simulink model "PMSM"  (R2024b)
settings: Solver=VariableStepAuto  StartTime=0.0  StopTime=3  RelTol=1e-3
values from neighbouring files (symbols this model uses):
  f_peak = 60    [PMSM_machine.m]
  J_total = 340e-6    (= 0.00034)    [PMSM_machine.m]
  Ls = 1365e-6    (= 0.001365)    [PMSM_machine.m]
  p = 2    [PMSM_machine.m]
  Psi_f = 0.166    [PMSM_machine.m]
  Rs = 0.416    [PMSM_machine.m]
  T_nom = 10    [PMSM_machine.m]
  t_ramp = 0.5    [PMSM_machine.m]
  U_peak = 60    [PMSM_machine.m]
libraries: mcbcontrolslib x4, simulink x2, eeTransforms x1
settings Model: Creator=chinm  LastModifiedBy=chinm

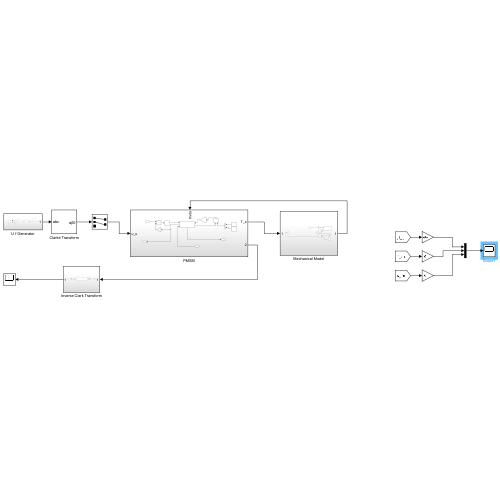
[thumbnail: Simulink's stored preview of the top-level diagram]
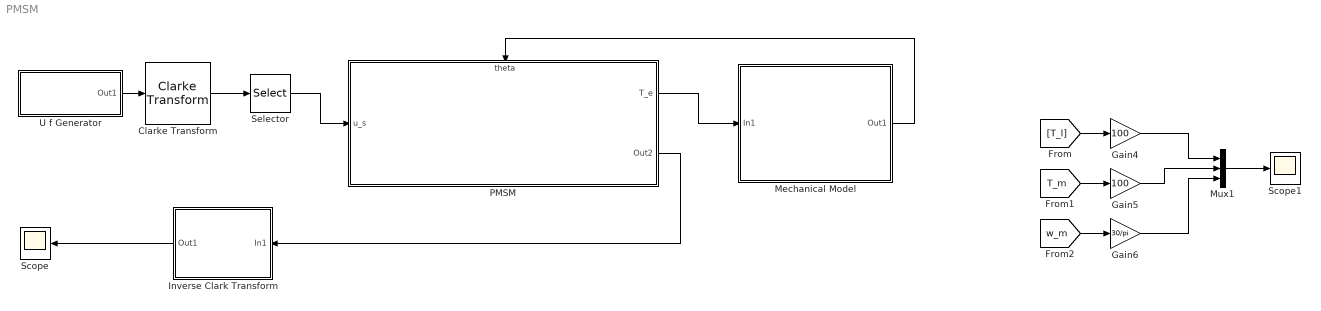
== system PMSM ==
  Clarke Transform : eeTransforms/Clarke Transform  PowerInvariant=off
      settings: LibrarySourceBlock=|
      | ee_sl_lib/Mathematical
      | Transforms/Clarke Transform
  Gain4 : Gain  Gain=100
  Gain5 : Gain  Gain=100
  Gain6 : Gain  Gain=30/pi
  Inverse Clark Transform : Subsystem
  Mechanical Model : Subsystem
  Mux1 : Mux  Inputs=3
  PMSM : Subsystem
      settings: PortSchema="{\"entries\":[{\"content\":{\"sides\":[{\"content\":{\"connectorIds\":[\"In1\"]},\"type\":\"ConnectorPlacement.EquallySpacedRectSide\",\"uuid\":\"4cb8065a-e5a2-415d-9e19-2924cebdfb7e\"},{\"content\":{\"connectorIds\":[\"Out1\",\"Out2\"],\"side\":\"RIGHT\"},\"type\":\"ConnectorPlacement.EquallySpacedRectSide\",\"uuid\":\"835c200d-c821-4b36-b5e5-04b20f8cfe15\"},{\"content\":{\"connectorIds\":[\"In2\"],\"side\":\"TOP\"},\"type\":\"ConnectorPlacement.EquallySpacedRectSide\",\"uuid\":\"b9320f7a-4b67-4ae1-910b-20da4fa2f11a\"}]},\"type\":\"ConnectorPlacement.EquallySpacedConnector\",\"uuid\":\"30be06dc-1f8c-4f24-82eb-4e3de7bbb2e4\"}],\"packageUris\":[\"http://schema.mathworks.com/mf0/Connector/R2020b\"],\"version\":\"1.0\"}"
  Scope : Scope
  Scope1 : Scope
  Selector : Selector  InputPortWidth=3  IndexOptions=Index vector (dialog)  Indices=[1 2]  OutputSizes=1
  U f Generator : Subsystem
  wires:
  U f Generator/1(Out1) -> Clarke Transform/1
  Clarke Transform/1 -> Selector/1
  Inverse Clark Transform/1(Out1) -> Scope/1
  [T_l] -> Gain4/1
  [T_m] -> Gain5/1
  [w_m] -> Gain6/1
  Mux1/1 -> Scope1/1
  Gain5/1 -> Mux1/2
  Gain4/1 -> Mux1/1
  Gain6/1 -> Mux1/3
  Selector/1 -> PMSM/1(u_s)
  PMSM/2(Out2) -> Inverse Clark Transform/1(In1)
  PMSM/1(T_e) -> Mechanical Model/1(In1)
  Mechanical Model/1(Out1) -> PMSM/2(theta)

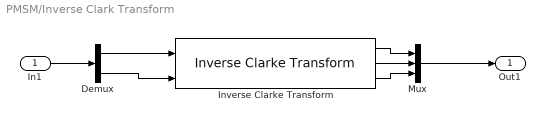
== system PMSM/Inverse Clark Transform ==
  In1 : Inport
  Demux : Demux  Outputs=2
  Inverse Clarke Transform : mcbcontrolslib/Inverse Clarke Transform  PhaseInput=Two inputs  EnPowerInv=off
      settings: LibrarySourceBlock=mcblib/Controls/Math Transforms/Inverse Clarke Transform
  Mux : Mux  Inputs=3
  Out1 : Outport
  wires:
  In1/1 -> Demux/1
  Demux/2 -> Inverse Clarke Transform/2
  Demux/1 -> Inverse Clarke Transform/1
  Inverse Clarke Transform/1 -> Mux/1
  Inverse Clarke Transform/2 -> Mux/2
  Inverse Clarke Transform/3 -> Mux/3
  Mux/1 -> Out1/1

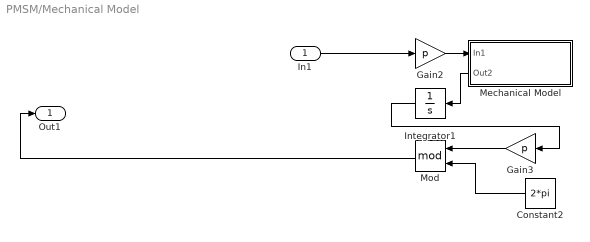
== system PMSM/Mechanical Model ==
  In1 : Inport
  Constant2 : Constant  Value=2*pi
  Gain2 : Gain  Gain=p
  Gain3 : Gain  Gain=p
  Integrator1 : Integrator
  Mechanical Model : Subsystem
      settings: PortSchema="{\"entries\":[{\"content\":{\"sides\":[{\"content\":{\"connectorIds\":[\"In1\",\"Out1\"]},\"type\":\"ConnectorPlacement.EquallySpacedRectSide\",\"uuid\":\"b4986fb2-c57d-4b73-a735-292653fff6d9\"},{\"content\":{\"side\":\"RIGHT\"},\"type\":\"ConnectorPlacement.EquallySpacedRectSide\",\"uuid\":\"9d0dc8a9-3fda-4760-870c-c4cad97d429b\"},{\"content\":{\"side\":\"TOP\"},\"type\":\"ConnectorPlacement.EquallySpacedRectSide\",\"uuid\":\"e1f646a3-730d-45a9-a867-cd53dcd150be\"}]},\"type\":\"ConnectorPlacement.EquallySpacedConnector\",\"uuid\":\"ab7f54df-393a-4b01-99b4-3432e63bf963\"}],\"packageUris\":[\"http://schema.mathworks.com/mf0/Connector/R2020b\"],\"version\":\"1.0\"}"
  Mod : Math  Operator=mod
  Out1 : Outport
  wires:
  Gain3/1 -> Mod/1
  Constant2/1 -> Mod/2
  Mechanical Model/1(Out2) -> Integrator1/1
  Integrator1/1 -> Gain3/1
  In1/1 -> Gain2/1
  Gain2/1 -> Mechanical Model/1(In1)
  Mod/1 -> Out1/1

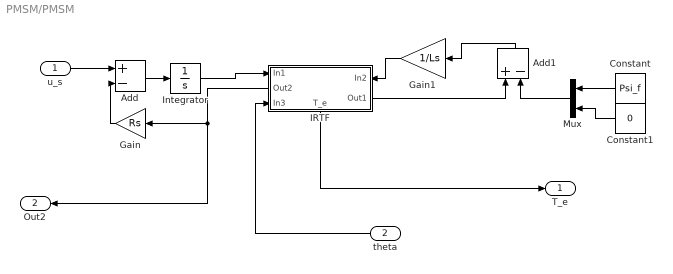
== system PMSM/PMSM ==
  u_s : Inport
  theta : Inport  Port=2
  Add : Sum  Inputs=+-
  Add1 : Sum  Inputs=+-
  Constant : Constant  Value=Psi_f
  Constant1 : Constant  Value=0
  Gain : Gain  Gain=Rs
  Gain1 : Gain  Gain=1/Ls
  IRTF : Subsystem
      settings: PortSchema="{\"entries\":[{\"content\":{\"sides\":[{\"content\":{\"connectorIds\":[\"In1\",\"Out3\",\"In2\"]},\"type\":\"ConnectorPlacement.EquallySpacedRectSide\",\"uuid\":\"b4986fb2-c57d-4b73-a735-292653fff6d9\"},{\"content\":{\"connectorIds\":[\"In3\",\"Out1\"],\"side\":\"RIGHT\"},\"type\":\"ConnectorPlacement.EquallySpacedRectSide\",\"uuid\":\"9d0dc8a9-3fda-4760-870c-c4cad97d429b\"},{\"content\":{\"side\":\"TOP\"},\"type\":\"ConnectorPlacement.EquallySpacedRectSide\",\"uuid\":\"e1f646a3-730d-45a9-a867-cd53dcd150be\"},{\"content\":{\"connectorIds\":[\"Out2\"],\"side\":\"BOTTOM\"},\"type\":\"ConnectorPlacement.EquallySpacedRectSide\",\"uuid\":\"c6f4b204-5ea6-4623-acea-3e4f968e6d8a\"}]},\"type\":\"ConnectorPlacement.EquallySpacedConnector\",\"uuid\":\"ab7f54df-393a-4b01-99b4-3432e63bf963\"}],\"packageUris\":[\"http://schema.mathworks.com/mf0/Connector/R2020b\"],\"version\":\"1.0\"}"
  Integrator : Integrator
  Mux : Mux  Inputs=2
  T_e : Outport
  Out2 : Outport  Port=2
  wires:
  IRTF/3(Out2) -> Out2/1, Gain/1
  Gain/1 -> Add/2
  u_s/1 -> Add/1
  Add/1 -> Integrator/1
  Integrator/1 -> IRTF/1(In1)
  Add1/1 -> Gain1/1
  Constant/1 -> Mux/1
  Constant1/1 -> Mux/2
  IRTF/1(Out1) -> Add1/1
  Mux/1 -> Add1/2
  Gain1/1 -> IRTF/3(In2)
  theta/1 -> IRTF/2(In3)
  IRTF/2(T_e) -> T_e/1

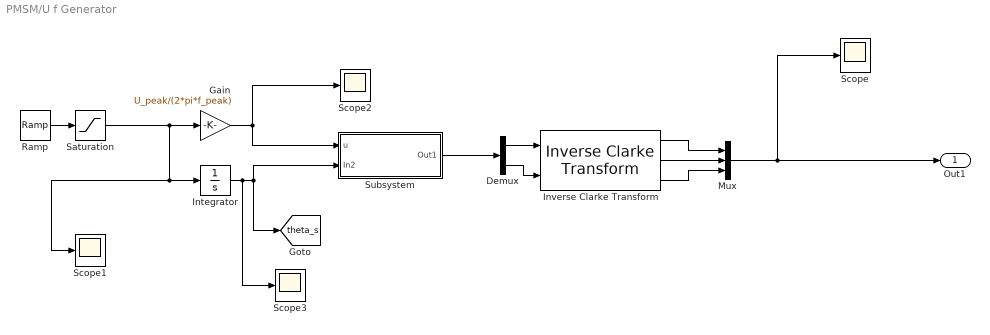
== system PMSM/U f Generator ==
  Demux : Demux  Outputs=2
  Gain : Gain  Gain=U_peak/(2*pi*f_peak)
  Integrator : Integrator  LimitOutput=on  WrappedStateUpperValue=2*pi  WrappedStateLowerValue=0  ZeroCross=off
  Inverse Clarke Transform : mcbcontrolslib/Inverse Clarke Transform  PhaseInput=Two inputs  EnPowerInv=off
      settings: LibrarySourceBlock=mcblib/Controls/Math Transforms/Inverse Clarke Transform
  Mux : Mux  Inputs=3
  Ramp : simulink/Sources/Ramp  slope=f_peak*2*pi/t_ramp  start=0  InitialOutput=0
  Saturation : Saturate  UpperLimit=2*pi*f_peak  LowerLimit=0
  Scope{,1..3} (4 alike) : Scope
  Subsystem : Subsystem
  Out1 : Outport
  tag scope: theta_s=global
  wires:
  Gain/1 -> Subsystem/1(u), Scope2/1
  Integrator/1 -> Scope3/1, Subsystem/2(In2), [theta_s]
  Demux/1 -> Inverse Clarke Transform/1
  Demux/2 -> Inverse Clarke Transform/2
  Inverse Clarke Transform/1 -> Mux/1
  Inverse Clarke Transform/2 -> Mux/2
  Inverse Clarke Transform/3 -> Mux/3
  Mux/1 -> Scope/1, Out1/1
  Ramp/1 -> Saturation/1
  Saturation/1 -> Integrator/1, Scope1/1, Gain/1
  Subsystem/1(Out1) -> Demux/1

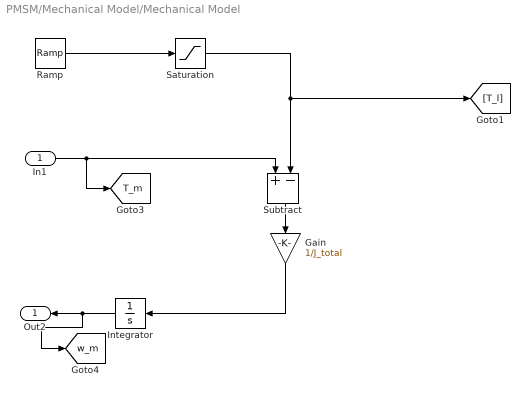
== system PMSM/Mechanical Model/Mechanical Model ==
  In1 : Inport
  Gain : Gain  Gain=1/J_total
  Integrator : Integrator
  Ramp : simulink/Sources/Ramp  slope=0.5*T_nom  start=1  InitialOutput=0
  Saturation : Saturate  UpperLimit=T_nom  LowerLimit=0
  Subtract : Sum  Inputs=+-
  Out2 : Outport
  tag scope: T_m=global, w_m=global
  wires:
  In1/1 -> Subtract/1, [T_m]
  Ramp/1 -> Saturation/1
  Saturation/1 -> [T_l], Subtract/2
  Subtract/1 -> Gain/1
  Gain/1 -> Integrator/1
  Integrator/1 -> [w_m], Out2/1

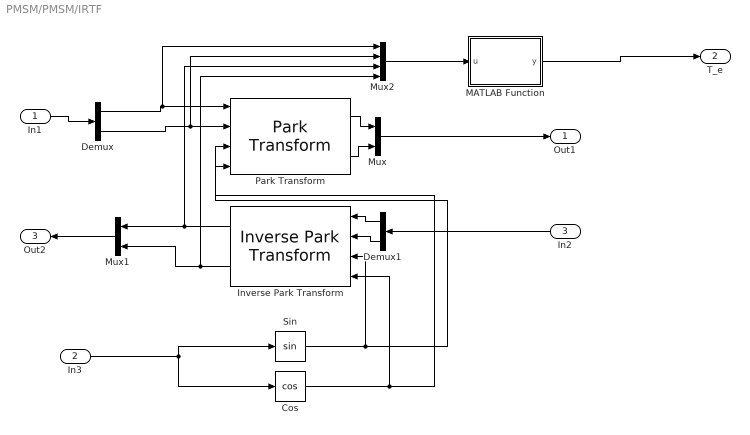
== system PMSM/PMSM/IRTF ==
  In1 : Inport
  In3 : Inport  Port=2
  In2 : Inport  Port=3
  Cos : Trigonometry  Operator=cos
  Demux : Demux  Outputs=2
  Demux1 : Demux  Outputs=2
  Inverse Park Transform : mcbcontrolslib/Inverse Park Transform  PhaseInput=Two inputs  AxisAlignment=D-axis  ThetaInput=Sine and Cosine electrical position  AngleInput=Per-unit  N_points=1024
      settings: LibrarySourceBlock=mcbhdllib/Controls/Math Transforms/Inverse Park Transform
  MATLAB Function : MATLAB Function  TreatAsAtomicUnit=on
  Mux : Mux  Inputs=2
  Mux1 : Mux  Inputs=2
  Mux2 : Mux
  Park Transform : mcbcontrolslib/Park Transform  PhaseInput=Two inputs  AxisAlignment=D-axis  ThetaInput=Sine and Cosine electrical position  AngleInput=Per-unit  N_points=1024
      settings: LibrarySourceBlock=mcblib/Controls/Math Transforms/Park Transform
  Sin : Trigonometry
  Out1 : Outport
  T_e : Outport  Port=2
  Out2 : Outport  Port=3
  wires:
  In1/1 -> Demux/1
  Demux/1 -> Mux2/1, Park Transform/1
  Demux/2 -> Mux2/2, Park Transform/2
  Park Transform/1 -> Mux/1
  Park Transform/2 -> Mux/2
  Mux/1 -> Out1/1
  In2/1 -> Demux1/1
  Demux1/1 -> Inverse Park Transform/1
  Demux1/2 -> Inverse Park Transform/2
  Inverse Park Transform/1 -> Mux2/3, Mux1/1
  Inverse Park Transform/2 -> Mux2/4, Mux1/2
  Mux1/1 -> Out2/1
  In3/1 -> Sin/1, Cos/1
  Sin/1 -> Park Transform/3, Inverse Park Transform/3
  Cos/1 -> Park Transform/4, Inverse Park Transform/4
  Mux2/1 -> MATLAB Function/1(u)
  MATLAB Function/1(y) -> T_e/1

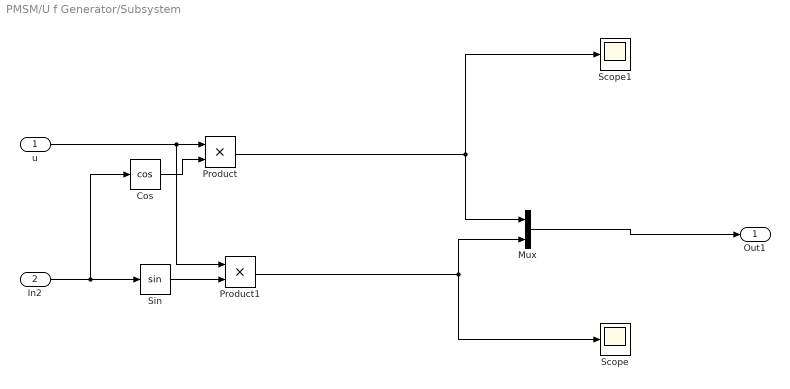
== system PMSM/U f Generator/Subsystem ==
  u : Inport
  In2 : Inport  Port=2
  Cos : Trigonometry  Operator=cos
  Mux : Mux  Inputs=2
  Product : Product
  Product1 : Product
  Scope : Scope
  Scope1 : Scope
  Sin : Trigonometry
  Out1 : Outport
  wires:
  Product/1 -> Scope1/1, Mux/1
  Product1/1 -> Mux/2, Scope/1
  Mux/1 -> Out1/1
  u/1 -> Product1/1, Product/1
  In2/1 -> Cos/1, Sin/1
  Cos/1 -> Product/2
  Sin/1 -> Product1/2

== matlab function PMSM/IRTF/MATLAB Function ==
  data: u input; y output
function y = fcn(u)

y = (u(1)*u(4)-u(2)*u(3))*3/2;
